simulink model "PD_ramp_and_step_input_final"  (R2022a)
settings: Solver=VariableStepAuto  StartTime=0.0  StopTime=10.0  RelTol=1e-3
libraries: slpidlib x1, simulink x1
settings Model: Creator=acer  LastModifiedBy=Electronica Care
settings SolverCC: AlgebraicLoopSolver=TrustRegion
settings DebuggingCC: SFMachineParentedDataDiag=warning  ArithmeticOperatorsInVariantConditions=warning
settings ModelReferenceCC: EnableRefExpFcnMdlSchedulingChecks=off
settings SFSimCC: CustomCodeUndefinedFunction=UseInterfaceOnly
settings RTWCC: Description=Generic Real-Time Target

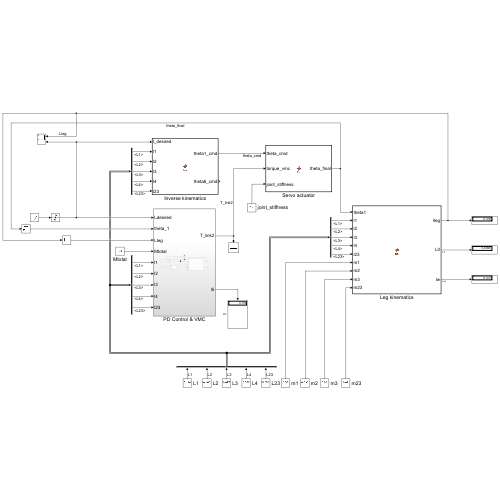
[thumbnail: Simulink's stored preview of the top-level diagram]
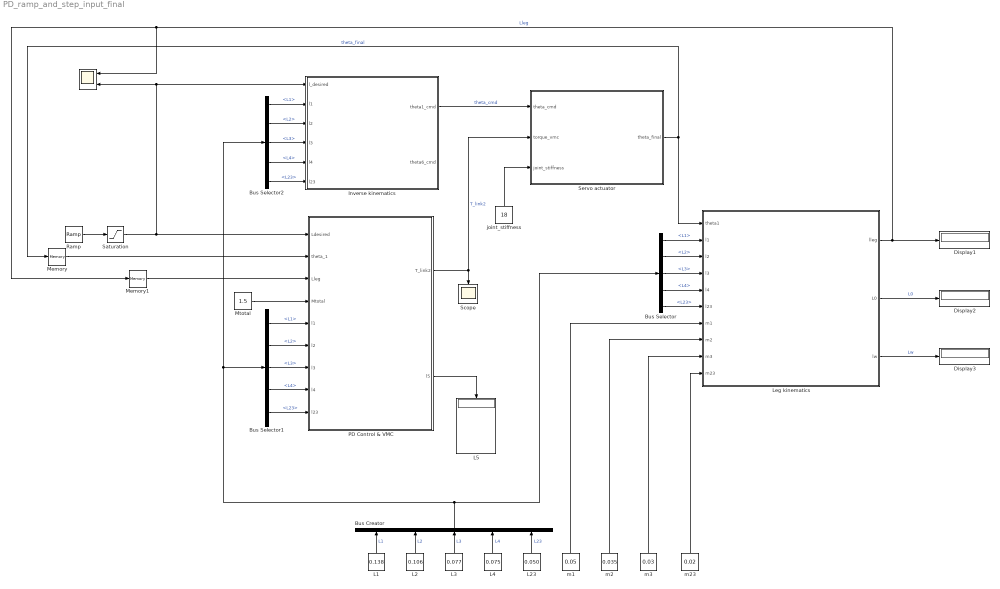
== system PD_ramp_and_step_input_final ==
  " " : Scope  NumInputPorts=2
  Bus Creator : BusCreator  Inputs=5
  Bus Selector : BusSelector  OutputSignals=L1,L2,L3,L4,L23
  Bus Selector1 : BusSelector  OutputSignals=L1,L2,L3,L4,L23
  Bus Selector2 : BusSelector  OutputSignals=L1,L2,L3,L4,L23
  Display1 : Display
  Display2 : Display
  Display3 : Display
  Inverse kinematics : MATLAB Function  TreatAsAtomicUnit=on
  L1 : Constant  Value=0.138
  L2 : Constant  Value=0.106
  L23 : Constant  Value=0.050
  L3 : Constant  Value=0.077
  L4 : Constant  Value=0.075
  L5 : Display
  Leg kinematics : MATLAB Function  TreatAsAtomicUnit=on
  Memory : Memory  InitialCondition=1
  Memory1 : Memory  InitialCondition=0.15
  Mtotal : Constant  Value=1.5
  PD Control & VMC : Subsystem
  Ramp : simulink/Sources/Ramp  slope=0.01  start=0  InitialOutput=0.1
  Saturation : Saturate  UpperLimit=0.18  LowerLimit=0.1
  Scope : Scope
  Servo actuator : MATLAB Function  TreatAsAtomicUnit=on
  joint_stiffness : Constant  Value=18
  m1 : Constant  Value=0.05
  m2 : Constant  Value=0.035
  m23 : Constant  Value=0.02
  m3 : Constant  Value=0.03
  wires:
  Servo actuator/1(theta_final) -> Memory/1, Leg kinematics/1(theta1)  "theta_final"
  PD Control & VMC/2(l5) -> L5/1
  PD Control & VMC/1(T_link2) -> Servo actuator/2(torque_vmc), Scope/1  "T_link2"
  Inverse kinematics/1(theta1_cmd) -> Servo actuator/1(theta_cmd)  "theta_cmd"
  joint_stiffness/1 -> Servo actuator/3(joint_stiffness)
  Leg kinematics/1(lleg) -> Memory1/1, " "/1, Display1/1  "Lleg"
  m1/1 -> Leg kinematics/7(m1)
  m2/1 -> Leg kinematics/8(m2)
  m3/1 -> Leg kinematics/9(m3)
  m23/1 -> Leg kinematics/10(m23)
  Leg kinematics/2(L0) -> Display2/1  "L0"
  Leg kinematics/3(lw) -> Display3/1  "Lw"
  Bus Selector/3 -> Leg kinematics/4(l3)  "<L3>"
  Bus Selector/2 -> Leg kinematics/3(l2)  "<L2>"
  Bus Selector/1 -> Leg kinematics/2(l1)  "<L1>"
  Bus Selector/4 -> Leg kinematics/5(l4)  "<L4>"
  Bus Selector/5 -> Leg kinematics/6(l23)  "<L23>"
  L3/1 -> Bus Creator/3  "L3"
  L2/1 -> Bus Creator/2  "L2"
  L1/1 -> Bus Creator/1  "L1"
  L4/1 -> Bus Creator/4  "L4"
  L23/1 -> Bus Creator/5  "L23"
  Bus Selector2/1 -> Inverse kinematics/2(l1)  "<L1>"
  Bus Selector2/2 -> Inverse kinematics/3(l2)  "<L2>"
  Bus Selector2/3 -> Inverse kinematics/4(l3)  "<L3>"
  Bus Selector2/4 -> Inverse kinematics/5(l4)  "<L4>"
  Bus Selector2/5 -> Inverse kinematics/6(l23)  "<L23>"
  Bus Selector1/1 -> PD Control & VMC/5(l1)  "<L1>"
  Bus Selector1/2 -> PD Control & VMC/6(l2)  "<L2>"
  Bus Selector1/3 -> PD Control & VMC/7(l3)  "<L3>"
  Bus Selector1/4 -> PD Control & VMC/8(l4)  "<L4>"
  Bus Selector1/5 -> PD Control & VMC/9(l23)  "<L23>"
  Bus Creator/1 -> Bus Selector/1, Bus Selector2/1, Bus Selector1/1
  Mtotal/1 -> PD Control & VMC/4(Mtotal)
  Memory1/1 -> PD Control & VMC/3(Lleg)
  Memory/1 -> PD Control & VMC/2(theta_1)
  Saturation/1 -> Inverse kinematics/1(l_desired), " "/2, PD Control & VMC/1(Ldesired)
  Ramp/1 -> Saturation/1

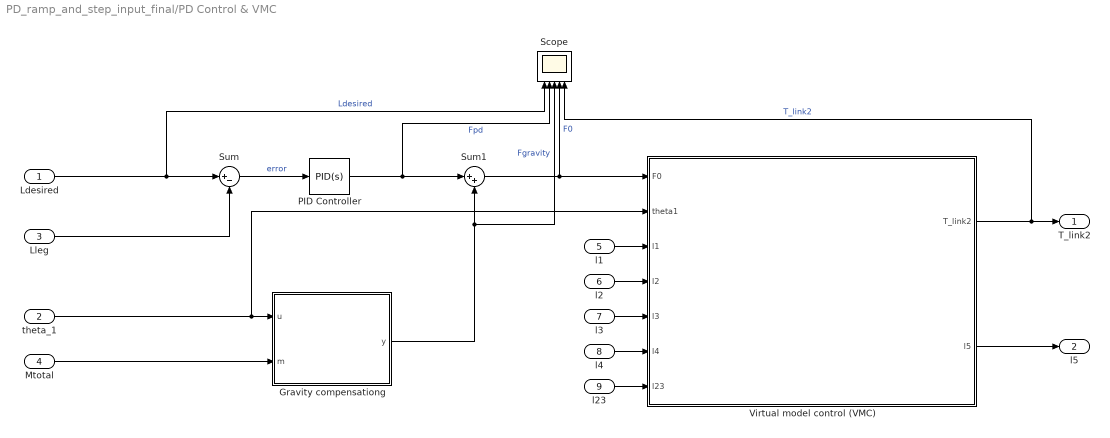
== system PD_ramp_and_step_input_final/PD Control & VMC ==
  Ldesired : Inport
  theta_1 : Inport  Port=2
  Lleg : Inport  Port=3
  Mtotal : Inport  Port=4
  l1 : Inport  Port=5
  l2 : Inport  Port=6
  l3 : Inport  Port=7
  l4 : Inport  Port=8
  l23 : Inport  Port=9
  Gravity compensationg : MATLAB Function  TreatAsAtomicUnit=on
  PID Controller : slpidlib/PID Controller  Controller=PID  Form=Parallel  TimeDomain=Continuous-time  UseExternalTs=off  SampleTime=-1  IntegratorMethod=Forward Euler  FilterMethod=Forward Euler  ControllerParametersSource=internal  P=0  I=2265.48971048851  UseKiTs=off  D=0  N=100  UseFilter=on  TunerSelectOption=Transfer Function Based (PID Tuner App)  InitialConditionSource=internal  InitialConditionForIntegrator=0  InitialConditionForFilter=0  DifferentiatorICPrevScaledInput=0  ExternalReset=none  TrackingMode=off  Kt=1  LimitOutput=off  SatLimitsSource=internal  UpperSaturationLimit=inf  LowerSaturationLimit=-inf  LinearizeAsGain=on  AntiWindupMode=none  Kb=1  POutMin=[]  POutMax=[]  IOutMin=[]  IOutMax=[]  DOutMin=[]  DOutMax=[]  NOutMin=[]  NOutMax=[]  SumOutMin=[]  SumOutMax=[]  SaturationOutMin=[]  SaturationOutMax=[]  PParamMin=[]  PParamMax=[]  IParamMin=[]  IParamMax=[]  DParamMin=[]  DParamMax=[]  NParamMin=[]  NParamMax=[]  KbParamMin=[]  KbParamMax=[]  KtParamMin=[]  KtParamMax=[]  KbOutMin=[]  KbOutMax=[]  KtOutMin=[]  KtOutMax=[]  IntegratorOutMin=[]  IntegratorOutMax=[]  FilterOutMin=[]  FilterOutMax=[]  SumI1OutMin=[]  SumI1OutMax=[]  SumI2OutMin=[]  SumI2OutMax=[]  SumI3OutMin=[]  SumI3OutMax=[]  SumI4OutMin=[]  SumI4OutMax=[]  SumDOutMin=[]  SumDOutMax=[]  DifferentiatorOutMin=[]  DifferentiatorOutMax=[]  FilterDiffOutCoefMin=[]  FilterDiffOutCoefMax=[]  ReciprocalOutMin=[]  ReciprocalOutMax=[]  SumDenOutMin=[]  SumDenOutMax=[]  SumNumOutMin=[]  SumNumOutMax=[]  DivideOutMin=[]  DivideOutMax=[]  UdiffTsProdOutMin=[]  UdiffTsProdOutMax=[]  NTsProdOutMin=[]  NTsProdOutMax=[]  UintegralTsProdOutMin=[]  UintegralTsProdOutMax=[]  UngainTsProdOutMin=[]  UngainTsProdOutMax=[]  IntegratorContinuousStateAttributes=''  IntegratorStateMustResolveToSignalObject=off  IntegratorRTWStateStorageClass=Auto  FilterContinuousStateAttributes=''  FilterStateMustResolveToSignalObject=off  FilterRTWStateStorageClass=Auto  ParallelPVariant=InternalParameters  IdealPVariant=Disabled  IVariant=InternalParameters  DVariant=InternalParameters  IntegratorVariant=Continuous  SatVariant=Disabled  AWVariant=Passthrough  PCopyVariant=Disabled  TRVariant=Disabled  FdbkBlocksVariant=Forward  IdealPFdbkVariant=Disabled  SatFdbkVariant=Disabled  DerivativeFilterVariant=ContFilter  NVariant=InternalParameters  NCopyVariant=Disabled  FilterICVariant=InternalICsFilter  IntegratorICVariant=InternalICs  ExternalResetVariant=Disabled  TRSumVariant=Passthrough  SumFdbkVariant=Disabled  SumVariant=Sum_PID  TsampFilterVariant=InternalTs  TsampNgainVariant=Passthrough  TsampIntegralVariant=Passthrough  ExternalSaturationOutDataTypeStr=Inherit: Same as second input  aMode=0
  Scope : Scope  NumInputPorts=5
  Sum : Sum  Inputs=|+-
  Sum1 : Sum  Inputs=|++
  Virtual model control (VMC) : MATLAB Function  TreatAsAtomicUnit=on
  T_link2 : Outport
  l5 : Outport  Port=2
  wires:
  l1/1 -> Virtual model control (VMC)/3(l1)
  l3/1 -> Virtual model control (VMC)/5(l3)
  Gravity compensationg/1(y) -> Scope/3, Sum1/2  "Fgravity"
  l23/1 -> Virtual model control (VMC)/7(l23)
  Lleg/1 -> Sum/2
  Sum/1 -> PID Controller/1  "error"
  theta_1/1 -> Virtual model control (VMC)/2(theta1), Gravity compensationg/1(u)
  Ldesired/1 -> Scope/1, Sum/1  "Ldesired"
  l2/1 -> Virtual model control (VMC)/4(l2)
  Sum1/1 -> Virtual model control (VMC)/1(F0), Scope/4  "F0"
  Virtual model control (VMC)/1(T_link2) -> Scope/5, T_link2/1  "T_link2"
  PID Controller/1 -> Scope/2, Sum1/1  "Fpd"
  l4/1 -> Virtual model control (VMC)/6(l4)
  Mtotal/1 -> Gravity compensationg/2(m)
  Virtual model control (VMC)/2(l5) -> l5/1

== matlab function PD_ramp_and_step_input_final/PD Control & VMC/Virtual model control (VMC) ==
  data: F0 input; T_link2 output; theta1 input; l1 input; l2 input; l3 input; l4 input; l23 input; l5 output
function [T_link2, l5] = fcn(F0, theta1, l1, l2, l3, l4, l23)

    l5 = sqrt(l2^2 + l4^2 - 2*l2*l4*cos(theta1 + pi/4));

    alpha_val = asin((l4 * sin(theta1 + pi/4)) / l5);
    
    cos_beta_arg = (l23^2 + l5^2 - l3^2) / (2 * l23 * l5);
    cos_beta_arg = max(min(cos_beta_arg, 1), -1);
    beta_val = acos(cos_beta_arg);

    J1 = l2 * cos(theta1) + l1 * cos(theta1 + alpha_val + beta_val);
    T_link2 = F0 * J1;

end

== matlab function PD_ramp_and_step_input_final/PD Control & VMC/Gravity compensationg ==
  data: u input; y output; m input
function y = fcn(u,m)

y = m*9.81*cos(u);
end

== matlab function PD_ramp_and_step_input_final/Inverse kinematics ==
  data: l_desired input; theta1_cmd output; l1 input; l2 input; l3 input; l4 input; l23 input; theta6_cmd output
function [theta1_cmd, theta6_cmd] = fcn(l_desired, l1, l2, l3, l4, l23)
    
    arg1 = (l_desired^2 + l2^2 - l1^2) / (2 * l_desired * l2);
    arg1 = max(min(arg1, 1), -1);
    theta1_cmd = asin(arg1);
    
    
    l5 = sqrt(l2^2 + l4^2 - 2*l2*l4*cos(theta1_cmd + pi/4));
    
    
    theta2 = asin((l4 * sin(theta1_cmd + pi/4)) / l5);
    
    
    arg3 = (l23^2 + l5^2 - l3^2) / (2 * l23 * l5);
    arg3 = max(min(arg3, 1), -1);
    theta3 = acos(arg3);
    
    
    theta4 = pi - theta1_cmd - theta2 - theta3;
    
    
    arg6 = (l5 * sin(theta3)) / l3;
    arg6 = max(min(arg6, 1), -1);
    theta6_cmd = asin(arg6) - theta4;
end

== matlab function PD_ramp_and_step_input_final/Servo actuator ==
  data: theta_cmd input; theta_final output; torque_vmc input; joint_stiffness input
function theta_final = fcn(theta_cmd, torque_vmc, joint_stiffness)

    delta_theta = torque_vmc / joint_stiffness;

    theta_final = theta_cmd + delta_theta;

end

== matlab function PD_ramp_and_step_input_final/Leg kinematics ==
  data: theta1 input; lleg output; l1 input; l2 input; l3 input; l4 input; l23 input; m1 input; m2 input; m3 input; m23 input; L0 output; lw output
function [lleg, L0, lw] = fcn(theta1, l1, l2, l3, l4, l23, m1, m2, m3, m23)
    
    l5 = sqrt(l2^2 + l4^2 - 2 * l2 * l4 * cos(theta1 + pi/4));
    
    arg_asin = (l4 * sin(theta1 + pi/4)) / l5;
    arg_asin = max(min(arg_asin, 1), -1); 
    theta2 = asin(arg_asin);
   
    arg_acos = (l23^2 + l5^2 - l3^2) / (2 * l23 * l5);
    arg_acos = max(min(arg_acos, 1), -1);
    theta3 = acos(arg_acos);
    
   
    theta4 = pi - theta1 - theta2 - theta3;
    theta5 = pi - theta4;
    
    arg_asin_theta6 = (l5 * sin(theta3)) / l3;
    arg_asin_theta6 = max(min(arg_asin_theta6, 1), -1);
    theta6 = asin(arg_asin_theta6) - theta4;
    
    lleg = l2 * sin(theta1) + l1 * sin(theta4);
    
    xc2 = (l2 * sin(theta1)) / 2;
    xc1 = l2 * sin(theta1) + (l1 * sin(theta5)) / 2;
    xc3 = -l4 * sin(pi/4) + (l3 * sin(theta6)) / 2;
    xc23 = l2 * sin(theta1) - (l23 * sin(theta4)) / 2;
    
    L0 = (m1*xc1 + m2*xc2 + m3*xc3 + m23*xc23) / (m1 + m2 + m3 + m23);
    
    lw = lleg - L0;
    
end
